simulink model "GNSS_Simulator"  (R2015b)
settings: Solver=VariableStepAuto  StartTime=0.0  StopTime=10.0  RelTol=1e-3
settings Model: Creator=scd2bp  LastModifiedBy=scd2bp

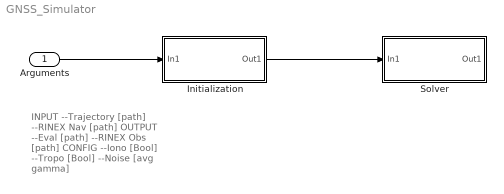
== system GNSS_Simulator ==
  note: INPUT
      | --Trajectory [path]
      | --RINEX Nav [path]
      |
      | OUTPUT
      | --Eval [path]
      | --RINEX Obs [path]
      |
      | CONFIG
      | --Iono [Bool]
      | --Tropo [Bool]
      | --Noise [avg gamma]
  Arguments : Inport
  Initialization : Subsystem
  Solver : Subsystem
  wires:
  Arguments/1 -> Initialization/1(In1)
  Initialization/1(Out1) -> Solver/1(In1)

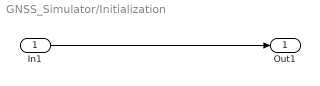
== system GNSS_Simulator/Initialization ==
  In1 : Inport
  Out1 : Outport
  wires:
  In1/1 -> Out1/1

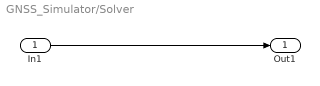
== system GNSS_Simulator/Solver ==
  In1 : Inport
  Out1 : Outport
  wires:
  In1/1 -> Out1/1
